simulink model "lab6_sim2"  (R2024a)
settings: Solver=VariableStepAuto  StartTime=0.0  StopTime=10.0  RelTol=1e-3
settings Model: Creator=ventus  LastModifiedBy=ventus

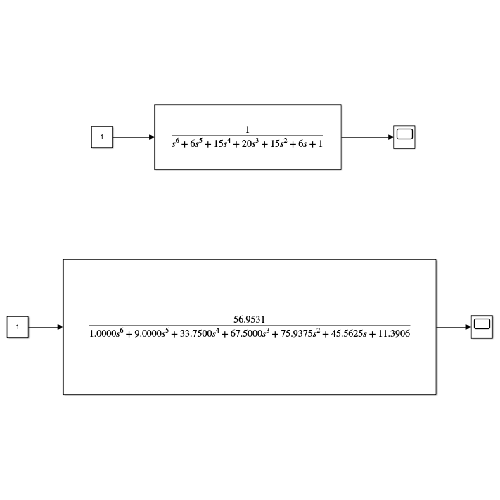
[thumbnail: Simulink's stored preview of the top-level diagram]
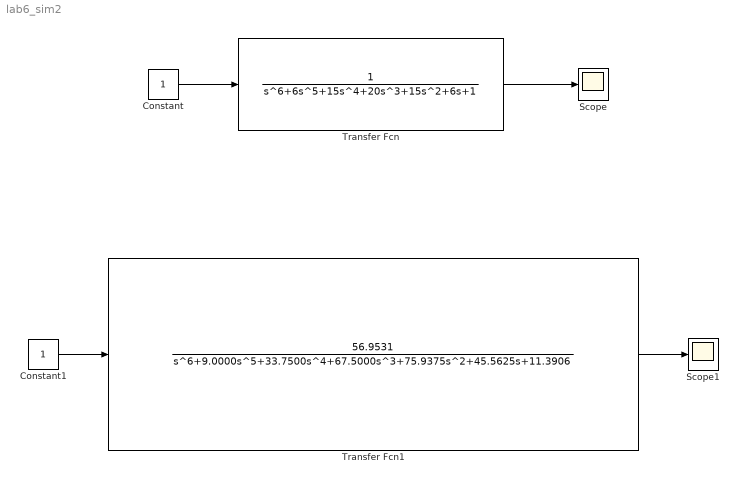
== system lab6_sim2 ==
  Constant : Constant
  Constant1 : Constant
  Scope : Scope
  Scope1 : Scope
  Transfer Fcn : TransferFcn  Denominator="[1     6    15    20    15     6     1]"
  Transfer Fcn1 : TransferFcn  Numerator=[56.9531]  Denominator=|
      | [1.0000
      |     9.0000
      |    33.7500
      |    67.5000
      |    75.9375
      |    45.5625
      |    11.3906]
  wires:
  Constant/1 -> Transfer Fcn/1
  Transfer Fcn/1 -> Scope/1
  Constant1/1 -> Transfer Fcn1/1
  Transfer Fcn1/1 -> Scope1/1
